simulink model "ADC_stateflow"  (R2020b)
settings: Solver=VariableStepAuto  StartTime=0.0  StopTime=5  RelTol=1e-3
values from neighbouring files (symbols this model uses):
  Cf = minimum_cap    [SAR_ADC.m]    (also in SNDRvsIdealSNDR.m; SNDRvsPowerIdeal.m; noiselessSNDRvsIdealSNDR.m)
  clk_period = 1/clk_freq    (= 0.000265731292517)    [SAR_ADC.m]    (also in SNDRvsIdealSNDR.m = 1/clk_freq; SNDRvsPowerIdeal.m = 1/clk_freq; noiselessSNDRvsIdealSNDR.m = 1/clk_freq)
  comparator_high_offset = 0.2*10e-4    (= 0.0002)    [SAR_ADC.m]    (also in SNDRvsIdealSNDR.m; SNDRvsPowerIdeal.m; noiselessSNDRvsIdealSNDR.m)
  comparator_low_offset = -.1*10e-4    (= -0.0001)    [SAR_ADC.m]    (also in SNDRvsIdealSNDR.m; SNDRvsPowerIdeal.m; noiselessSNDRvsIdealSNDR.m)
  comparator_offset_on = non_idealities_on    (= 1)    [SAR_ADC.m]    (also in SNDRvsIdealSNDR.m = 0; SNDRvsPowerIdeal.m = 0; noiselessSNDRvsIdealSNDR.m = 0)
  k = 1.38064852e-23    [SAR_ADC.m]    (also in SNDRvsIdealSNDR.m; SNDRvsPowerIdeal.m; noiselessSNDRvsIdealSNDR.m)
  number_of_bits = 6    [SAR_ADC.m]    (also in SNDRvsIdealSNDR.m = 1+i; SNDRvsPowerIdeal.m = 1+i; noiselessSNDRvsIdealSNDR.m = 1+i)
  sample_time_jitter = 16e-12    (= 1.6e-11)    [SAR_ADC.m]    (also in SNDRvsIdealSNDR.m; SNDRvsPowerIdeal.m; noiselessSNDRvsIdealSNDR.m)
  sampling_gain = Cs/Cf    [SAR_ADC.m]    (also in SNDRvsIdealSNDR.m; SNDRvsPowerIdeal.m; noiselessSNDRvsIdealSNDR.m)
  sampling_jitter_on = non_idealities_on    (= 1)    [SAR_ADC.m]    (also in SNDRvsIdealSNDR.m; SNDRvsPowerIdeal.m = 0; noiselessSNDRvsIdealSNDR.m = 0)
  sine_amplitude = .001    (= 0.001)    [SAR_ADC.m]    (also in SNDRvsIdealSNDR.m; SNDRvsPowerIdeal.m; noiselessSNDRvsIdealSNDR.m)
  sine_bias = 0    [SAR_ADC.m]    (also in SNDRvsIdealSNDR.m; SNDRvsPowerIdeal.m; noiselessSNDRvsIdealSNDR.m)
  sine_frequency_rad = 2*pi*sine_freq    (= 1256.63706144)    [SNDRvsIdealSNDR.m]    (also in SNDRvsPowerIdeal.m; noiselessSNDRvsIdealSNDR.m)
  switch_noise_on = non_idealities_on    (= 1)    [SAR_ADC.m]    (also in SNDRvsIdealSNDR.m; SNDRvsPowerIdeal.m = 0; noiselessSNDRvsIdealSNDR.m = 0)
  T = 293    [SAR_ADC.m]    (also in SNDRvsIdealSNDR.m; SNDRvsPowerIdeal.m; noiselessSNDRvsIdealSNDR.m)
  Vref = 2    [SAR_ADC.m]    (also in SNDRvsIdealSNDR.m; SNDRvsPowerIdeal.m; noiselessSNDRvsIdealSNDR.m)
libraries: simulink_extras x1, simulink x1
settings Model: SnapshotInterval=1  Creator=mac  LastModifiedBy=mac
settings DataIOCC: SaveFormat=Structure
settings DebuggingCC: UnderSpecifiedDimensionMsg=warning

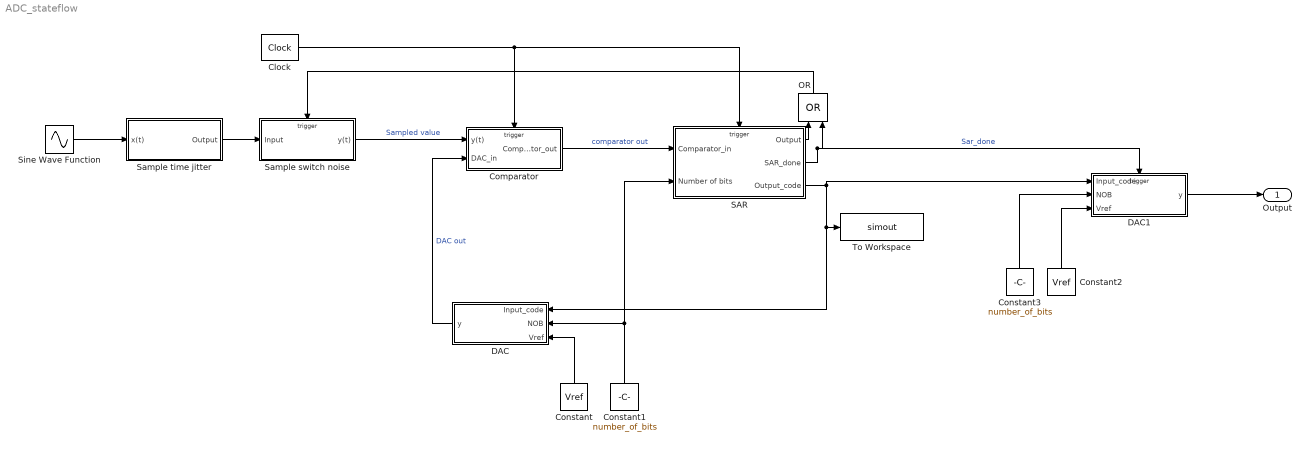
== system ADC_stateflow ==
  Clock : simulink_extras/Flip Flops/Clock  period=clk_period
  Comparator : Subsystem  TreatAsAtomicUnit=on
  Constant : Constant  Value=Vref
  Constant1 : Constant  Value=number_of_bits
  Constant2 : Constant  Value=Vref
  Constant3 : Constant  Value=number_of_bits
  DAC : Subsystem  TreatAsAtomicUnit=on
  DAC1 : Subsystem
  OR : Logic  Operator=OR  IconShape=distinctive  AllPortsSameDT=off  OutDataTypeStr=boolean
  SAR : Subsystem  TreatAsAtomicUnit=on
  Sample switch noise : Subsystem  TreatAsAtomicUnit=on
  Sample time jitter : Subsystem
  Sine Wave Function : Sin  Amplitude=sine_amplitude  Bias=sine_bias  Frequency=sine_frequency_rad  SampleTime=0
  To Workspace : ToWorkspace  VariableName=simout  SaveFormat=Structure  SampleTime=-1
  Output : Outport
  wires:
  Constant/1 -> DAC/3(Vref)
  Constant1/1 -> DAC/2(NOB), SAR/2(Number of bits)
  SAR/3(Output_code) -> To Workspace/1, DAC/1(Input_code), DAC1/1(Input_code)
  Constant2/1 -> DAC1/3(Vref)
  Constant3/1 -> DAC1/2(NOB)
  Clock/1 -> SAR/Trigger, Comparator/Trigger
  Sample switch noise/1(y(t)) -> Comparator/1(y(t))  "Sampled value"
  SAR/2(SAR_done) -> OR/2, DAC1/Trigger  "Sar_done"
  DAC/1(y) -> Comparator/2(DAC_in)  "DAC out"
  Comparator/1(Comparator_out) -> SAR/1(Comparator_in)  "comparator out"
  DAC1/1(y) -> Output/1
  OR/1 -> Sample switch noise/Trigger
  SAR/1(Output) -> OR/1
  Sample time jitter/1(Output) -> Sample switch noise/1(Input)
  Sine Wave Function/1 -> Sample time jitter/1(x(t))

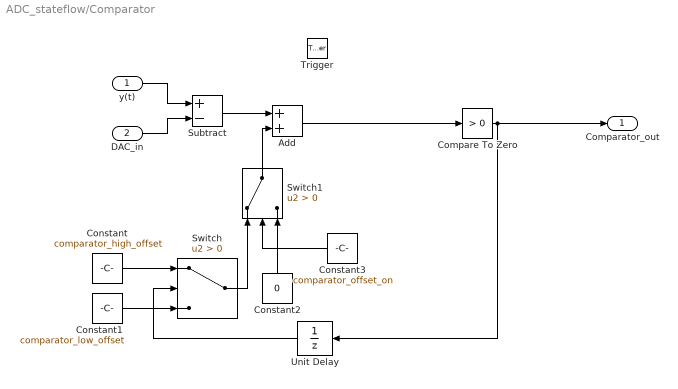
== system ADC_stateflow/Comparator ==
  y(t) : Inport
  DAC_in : Inport  Port=2
  Trigger : TriggerPort  VariantControl=Variant
  Add : Sum
  Compare To Zero : simulink/Logic and Bit Operations/Compare To Zero  relop=>  OutDataTypeStr=boolean
  Constant : Constant  Value=comparator_high_offset
  Constant1 : Constant  Value=comparator_low_offset
  Constant2 : Constant  Value=0
  Constant3 : Constant  Value=comparator_offset_on
  Subtract : Sum  Inputs=+-
  Switch : Switch  Criteria=u2 > Threshold
  Switch1 : Switch  Criteria=u2 > Threshold
  Unit Delay : UnitDelay  SampleTime=-1  HasFrameUpgradeWarning=on
  Comparator_out : Outport
  wires:
  Switch/1 -> Switch1/1
  Subtract/1 -> Add/1
  Constant/1 -> Switch/1
  Constant2/1 -> Switch1/3
  y(t)/1 -> Subtract/1
  Add/1 -> Compare To Zero/1
  Switch1/1 -> Add/2
  Compare To Zero/1 -> Unit Delay/1, Comparator_out/1
  Constant3/1 -> Switch1/2
  Unit Delay/1 -> Switch/2
  Constant1/1 -> Switch/3
  DAC_in/1 -> Subtract/2

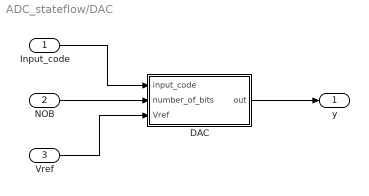
== system ADC_stateflow/DAC ==
  Input_code : Inport
      settings: VarSizeSig=Yes
  NOB : Inport  Port=2
  Vref : Inport  Port=3
  DAC : MATLAB Function  TreatAsAtomicUnit=on
  y : Outport
  wires:
  NOB/1 -> DAC/2(number_of_bits)
  Vref/1 -> DAC/3(Vref)
  DAC/1(out) -> y/1
  Input_code/1 -> DAC/1(input_code)

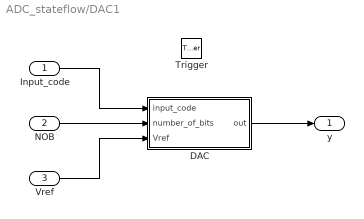
== system ADC_stateflow/DAC1 ==
  Input_code : Inport
  NOB : Inport  Port=2
  Vref : Inport  Port=3
  Trigger : TriggerPort  VariantControl=Variant  PortDimensions=1
  DAC : MATLAB Function  TreatAsAtomicUnit=on
  y : Outport
  wires:
  Input_code/1 -> DAC/1(input_code)
  DAC/1(out) -> y/1
  NOB/1 -> DAC/2(number_of_bits)
  Vref/1 -> DAC/3(Vref)

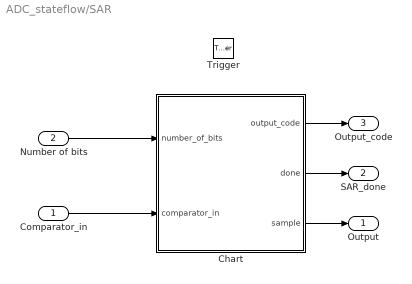
== system ADC_stateflow/SAR ==
  Comparator_in : Inport  LatchByDelayingOutsideSignal=on
  Number of bits : Inport  Port=2
  Trigger : TriggerPort  VariantControl=Variant
  Chart : Stateflow chart  TreatAsAtomicUnit=on
  Output : Outport
  SAR_done : Outport  Port=2
  Output_code : Outport  Port=3  InitialOutput=zeros(number_of_bits,1)
      settings: VarSizeSig=Yes
  wires:
  Number of bits/1 -> Chart/1(number_of_bits)
  Chart/1(output_code) -> Output_code/1
  Comparator_in/1 -> Chart/2(comparator_in)
  Chart/2(done) -> SAR_done/1
  Chart/3(sample) -> Output/1

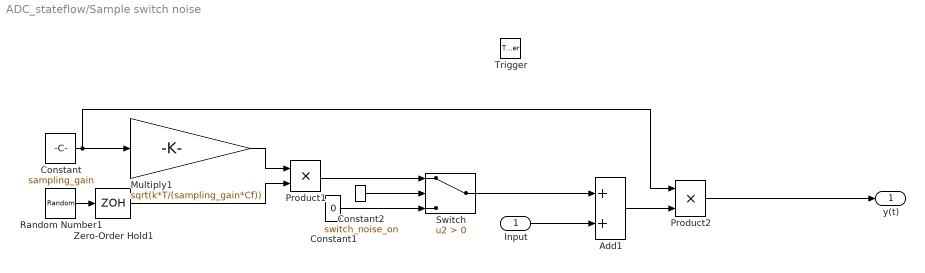
== system ADC_stateflow/Sample switch noise ==
  Input : Inport
  Trigger : TriggerPort  VariantControl=Variant
  Add1 : Sum
  Constant : Constant  Value=sampling_gain
  Constant1 : Constant  Value=0
  Constant2 : Constant  Value=switch_noise_on
  Multiply1 : Gain  Gain=sqrt(k*T/(sampling_gain*Cf))  OutDataTypeStr=Inherit: Same as input
  Product1 : Product
  Product2 : Product
  Random Number1 : RandomNumber
  Switch : Switch  Criteria=u2 > Threshold
  Zero-Order Hold1 : ZeroOrderHold  SampleTime=-1
  y(t) : Outport
  wires:
  Product2/1 -> y(t)/1
  Random Number1/1 -> Zero-Order Hold1/1
  Multiply1/1 -> Product1/1
  Add1/1 -> Product2/2
  Constant/1 -> Product2/1, Multiply1/1
  Constant2/1 -> Switch/2
  Constant1/1 -> Switch/3
  Product1/1 -> Switch/1
  Zero-Order Hold1/1 -> Product1/2
  Switch/1 -> Add1/1
  Input/1 -> Add1/2

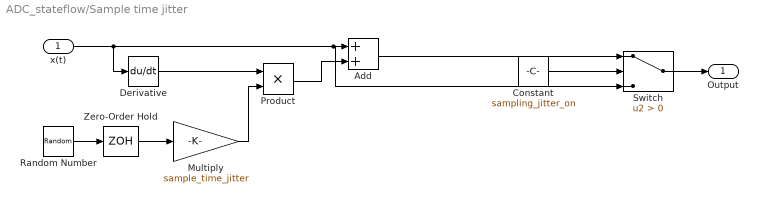
== system ADC_stateflow/Sample time jitter ==
  x(t) : Inport
  Add : Sum
  Constant : Constant  Value=sampling_jitter_on
  Derivative : Derivative
  Multiply : Gain  Gain=sample_time_jitter
  Product : Product
  Random Number : RandomNumber  SampleTime=clk_period
  Switch : Switch  Criteria=u2 > Threshold
  Zero-Order Hold : ZeroOrderHold  SampleTime=-1
  Output : Outport
  wires:
  Random Number/1 -> Zero-Order Hold/1
  x(t)/1 -> Add/1, Switch/3, Derivative/1
  Zero-Order Hold/1 -> Multiply/1
  Product/1 -> Add/2
  Derivative/1 -> Product/1
  Multiply/1 -> Product/2
  Switch/1 -> Output/1
  Add/1 -> Switch/1
  Constant/1 -> Switch/2

== matlab function ADC_stateflow/DAC1/DAC ==
  data: input_code input size=number_of_bits; out output double size=1; number_of_bits input; Vref input
function out = fcn(input_code, number_of_bits, Vref)
out = Vref*bi2de(input_code.', 'left-msb')/(2^(number_of_bits));
end

== matlab function ADC_stateflow/DAC/DAC ==
  data: input_code input size=number_of_bits; out output double size=1; number_of_bits input; Vref input
function out = fcn(input_code, number_of_bits, Vref)
out = Vref/(2^number_of_bits)*(bi2de(input_code.', 'left-msb'));
end

== stateflow chart ADC_stateflow/SAR/Chart ==
  settings: sampleTime=clk_period
  state SAR
    cycle=cycle+1;
    output_code(cycle-1, 1)=comparator_in;
    done=false;
    output_code(cycle, 1) = 1;
  state Initial
    done=false;
    output_code = zeros(number_of_bits, 1);
    output_code(1,1) = 1;
    cycle=1;
    sample=false;
  state AlmostDone
    done=false;
    output_code(number_of_bits-1,1) = comparator_in;
    output_code(number_of_bits,1) = 1;
  state Start
    sample = true;
    done = false;
    output_code = zeros(number_of_bits, 1);
  state Done
    done=true;
    output_code(number_of_bits, 1) = comparator_in;
  Initial -> AlmostDone [order 2] : [cycle==number_of_bits-1]
  (default) -> Start
  Initial -> SAR [order 1] : [cycle<number_of_bits-1]
  SAR -> AlmostDone [order 1] : [cycle==number_of_bits-1]
  Start -> Initial
  AlmostDone -> Done
  Done -> Initial
  Initial -> Done [order 3] : [number_of_bits==1]
  SAR -> SAR [order 2] : [cycle<(number_of_bits-1)]
  data: cycle local double size=1; output_code output size=number_of_bits; number_of_bits input; comparator_in input; done output; sample output
